simulink model "Quad3d_depth_semantic_segmentation"  (R2024b)
settings: Solver=VariableStepAuto  StartTime=0.0  StopTime=10.0  RelTol=1e-3
undefined symbols (not defined in the file): Sim3dSensor
libraries: simulink x2, sim3dcameralib x1, sim3dlib x1, uavsim3dlib x1
settings Model: Creator=Adi

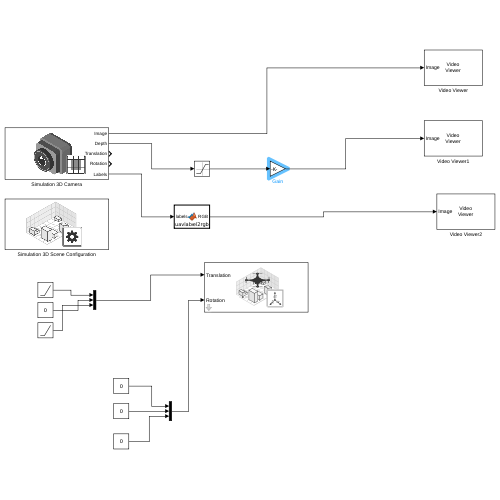
[thumbnail: Simulink's stored preview of the top-level diagram]
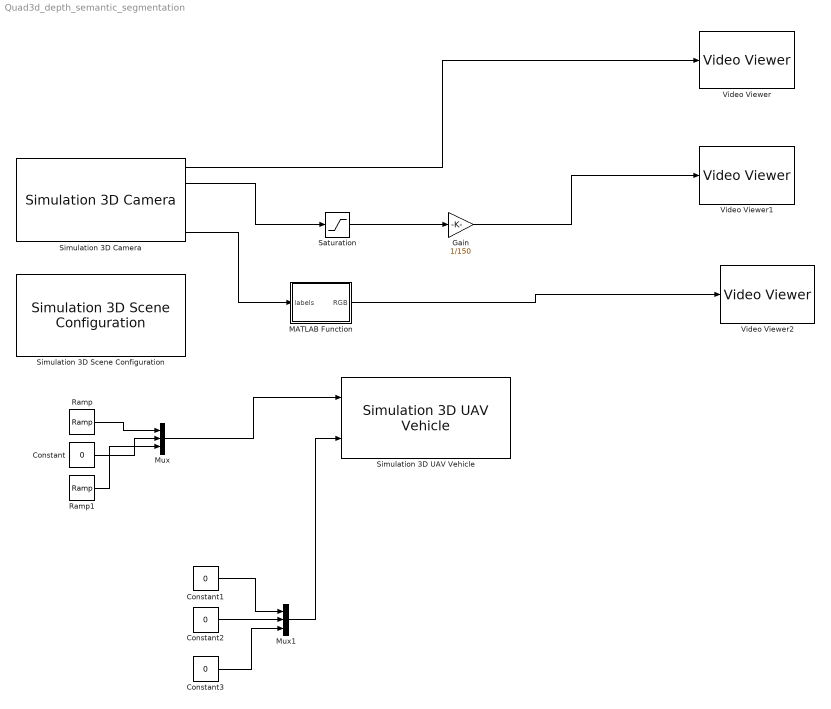
== system Quad3d_depth_semantic_segmentation ==
  Constant{,1..3} (4 alike) : Constant  Value=0
  Gain : Gain  Gain=1/150
  MATLAB Function : MATLAB Function  TreatAsAtomicUnit=on
  Mux : Mux  Inputs=3
  Mux1 : Mux  Inputs=3
  Ramp : simulink/Sources/Ramp  slope=1  start=0  InitialOutput=0
  Ramp1 : simulink/Sources/Ramp  slope=1  start=0  InitialOutput=0
  Saturation : Saturate  UpperLimit=150  LowerLimit=0
  Simulation 3D Camera : sim3dcameralib/Simulation 3D Camera  Priority=1  sensorTag=Sim3dSensor�  sensorId=1  sensorName=Sim3dSensor�  vehTagList={'Scene Origin';'SimulinkVehicle1'}  vehTag=SimulinkVehicle1  mountLoc=Origin  offsetFlag=on  tmountOffset=[0, 0, 0]  extTmount=off  rmountOffset=[0, 0, 0]  extRmount=off  FocalLength=[1109, 1109]  OpticalCenter=[640, 360]  ImageSize=[720, 1280]  RadialDistortion=[0, 0]  TangentialDistortion=[0, 0]  SensorSkew=0  DepthOutportEnabled=on  SemanticOutportEnabled=on  TransformOutportEnabled=on  SampleTime=-1  mountPoint=[0 0 0]  mountOrientation=[0 0 0]  aMode=4  ID=1
      settings: LibrarySourceBlock=uavsim3dlib/Simulation 3D Camera
  Simulation 3D Scene Configuration : sim3dlib/Simulation 3D Scene Configuration  Priority=0  ProjectFormat=Default Scenes  SceneDesc=US city block  ProjectName=/MATLAB/toolbox/shared/sim3d_projects/automotive_project_linux/UE/LinuxNoEditor/VehicleSimulation.sh  ScenePath=/Game/Maps/USCityBlock  EnableOpenDRIVE=off  vehTagList={'Custom';'Scene Origin';'SimulinkVehicle1'}  vehTag=Scene Origin  FreeCameraInitialTranslation=[0, 0, 0]  FreeCameraDefaultInitialTranslation=[-6, 0, 2]  FreeCameraInitialRotation=[0, 0, 0]  FreeCameraDefaultInitialRotation=[0, -15, 0]  OpVisEn=off  Ts=1/60  EnableWindow=on  EnableRemoteAccess=off  EnableWeather=off  SunAzimuth=90  SunAltitude=40.0  EnableGeospatialSun=off  Latitude=0  Longitude=0  Date=2023-01-01  Time=10:30:00  GeoTimeZone=-5.0  SunDaylightSaving=off  wind=1  clouds=10  EnableVolumetricClouds=off  CloudCoverage=0  CloudAltitude=6  fog=0  rain=0  RaindropsEffect=off  SnowDensity=0  EnableGeospatial=off  UseTrueOrigin=off  OriginHeight=200  OriginLatitude=40.744652  OriginLongitude=-73.988864  MapStyle=Aerial  AdditionalAssetIDs=[]  UseAdvancedSunSky=off  SolarTime=11  TimeZone=-5  Day=21  Month=9  Year=2022  UseDaylightSavingTime=on  DSTStartDay=10  DSTStartMonth=3  DSTEndDay=3  DSTEndMonth=11  DSTSwitchHour=2  sensorTag=MainCamera1  sensorId=1  sensorName=MainCamera1  mountLoc=Origin  offsetFlag=off  tmountOffset=[0, 0, 0]  rmountOffset=[0, 0, 0]  HorizontalResolution=1280  VerticalResolution=720  HorizontalFOV=60  mountPoint=[0 0 0]  mountOrientation=[0 0 0]  aMode=4  ID=1  GeoTrigger=Inactive
      settings: LibrarySourceBlock=uavsim3dlib/Simulation 3D Scene Configuration
  Simulation 3D UAV Vehicle : uavsim3dlib/Simulation 3D UAV Vehicle  Priority=-1  Mesh=Quadrotor  MeshPath=/MathWorksUAVContent/UAVs/HexaRotorUAV/HexaRotor.HexaRotor  Color=Black  ActorName=SimulinkVehicle1  UseGlobalFrame=off  InitialTranslation=[0 0 0]  InitialRotation=[0 0 0]  InitialTranslationGlobal=[0 0 0]  InitialGeoOrigin=[0 0 0]  InitialRotationGlobal=[0 0 0]  SampleTime=-1  ActorType=SimulinkVehicle  ID=1  aMode=4  ActorTag=SimulinkVehicle1
  Video Viewer : VideoViewer  FigPos=[860.333333333333 654.666666666667 418 304]
  Video Viewer1 : VideoViewer  FigPos=[117.666666666667 478 418 304]
  Video Viewer2 : VideoViewer  FigPos=[113.666666666667 857.333333333333 418 304]
  wires:
  Ramp/1 -> Mux/1
  Constant/1 -> Mux/2
  Ramp1/1 -> Mux/3
  Constant1/1 -> Mux1/1
  Constant2/1 -> Mux1/2
  Constant3/1 -> Mux1/3
  Mux/1 -> Simulation 3D UAV Vehicle/1
  Mux1/1 -> Simulation 3D UAV Vehicle/2
  Simulation 3D Camera/1 -> Video Viewer/1
  Simulation 3D Camera/2 -> Saturation/1
  Saturation/1 -> Gain/1
  Gain/1 -> Video Viewer1/1
  Simulation 3D Camera/5 -> MATLAB Function/1(labels)
  MATLAB Function/1(RGB) -> Video Viewer2/1

== matlab function Quad3d_depth_semantic_segmentation/MATLAB Function ==
  data: labels input; RGB output
function RGB = uavlabel2rgb(labels)
coder.extrinsic('label2rgb');
RGB=coder.nullcopy(zeros(size(labels,1),size(labels,2),3,class(labels)));
cmap=sim3dColormap;
RGB=label2rgb(labels,cmap);
end
 
 
function cmap = sim3dColormap
% Define colormap for object labels used in 3D simulation environment.
 
cmap = [
128 0 0     % Label 1: Building
0 0 0       % Label 2: Not used
72 0 90     % Label 3: Other
0 0 0       % Label 4: Not used
192 192 192 % Label 5: Pole
128 0 128   % Label 6: Lane marking
128 64 128  % Label 7: Roads
60 40 222   % Label 8: Sidewalk
128 128 0   % Label 9: Vegetation
64 0 128    % Label 10: Vehicle
0 0 0       % Label 11: Not used
192 128 128 % Label 12: Generic traffic signs
192 128 128 % Label 13: Stop sign
192 128 128 % Label 14: Yield sign
192 128 128 % Label 15: Speed limit sign
192 128 128 % Label 16: Weight limit sign
0 0 0       % Label 17: Not used
0 0 0       % Label 18: Not used
192 128 128 % Label 19: Left and right arrow warning sign
192 128 128 % Label 20: Left chevron warning sign
192 128 128 % Label 21: Right chevron warning sign
0 0 0       % Label 22: Not used
192 128 128 % Label 23: Right one-way sign
0 0 0       % Label 24: Not used
192 128 128 % Label 25: School bus only sign
0 0 0       % Label 26: Not used
0 0 0       % Label 27: Not used
0 0 0       % Label 28: Not used
0 0 0       % Label 29: Not used
0 0 0       % Label 30: Not used
0 0 0       % Label 31: Not used
0 0 0       % Label 32: Not used
0 0 0       % Label 33: Not used
0 0 0       % Label 34: Not used
0 0 0       % Label 35: Not used
0 0 0       % Label 36: Not used
0 0 0       % Label 37: Not used
0 0 0       % Label 38: Not used
192 128 128 % Label 39: Crosswalk sign
0 0 0       % Label 40: Not used
192 128 128 % Label 41: Traffic signal
192 128 128 % Label 42: Curve right warning sign
192 128 128 % Label 43: Curve left warning sign
192 128 128 % Label 44: Up right arrow warning sign
0 0 0       % Label 45: Not used
0 0 0       % Label 46: Not used
0 0 0       % Label 47: Not used
192 128 128 % Label 48: Railroad crossing sign
192 128 128 % Label 49: Street sign
192 128 128 % Label 50: Roundabout warning sign
192 128 128 % Label 51: Fire hydrant
192 128 128 % Label 52: Exit sign
192 128 128 % Label 53: Bike lane sign
0 0 0       % Label 54: Not used
0 0 0       % Label 55: Not used
0 0 0       % Label 56: Not used
128 128 128 % Label 57: Sky
60 40 222   % Label 58: Curb
60 40 222   % Label 59: Flyover ramp
60 40 222   % Label 60: Road guard rail
0 0 0       % Label 61: Not used
0 0 0       % Label 62: Not used
0 0 0       % Label 63: Not used
0 0 0       % Label 64: Not used
0 0 0       % Label 65: Not used
0 0 0       % Label 66: Not used
240 150 25  % Label 67: Deer
0 0 0       % Label 68: Not used
0 0 0       % Label 69: Not used
0 0 0       % Label 70: Not used
150 50 15   % Label 71: Barricade
0 128 192   % Label 72: Motorcycle
];
 
% Normalize colormap to the range [0, 1].
cmap = cmap ./ 255;
 
end
